simulink library "util_generic_model_lib"  (R2016b)
settings: Solver=ode45  StartTime=0.0  StopTime=10.0  RelTol=1e-3  EnableMultiTasking=on
undefined symbols (not defined in the file): abp_impeller_diameter, abp_impeller_speed2pwm, abp_nozzle_flap_count, abp_nozzle_flap_length, abp_nozzle_gear_ratio, abp_nozzle_intake_height, abp_nozzle_min_open_angle, abp_P_CG_B_B_error, abp_PM1_discharge_coeff, abp_pm1_impeller_orientation, abp_PM1_nozzle_orientations, abp_PM1_nozzle_widths, abp_PM1_P_nozzle_B_B, abp_pm1_zero_thrust_area, astrobee_time_step_size, bmp_PM1_impeller_orientation_error, bpm_imp_cmd_filt_den, bpm_imp_cmd_filt_num, bpm_imp_ctl_filt_n, bpm_imp_ctl_kd, bpm_imp_ctl_ki, bpm_imp_ctl_kp, bpm_imp_ctl_ts, bpm_imp_max_voltage, bpm_imp_motor_friction_coeff, bpm_imp_motor_r, bpm_imp_motor_speed_k, bpm_imp_motor_torque_k, bpm_imp_speed_filt_den, bpm_imp_speed_filt_num, bpm_impeller_inertia, bpm_impeller_inertia_error, bpm_impeller_init_speed, bpm_lookup_Cdp_data, bpm_lookup_totalarea_breakpoints, bpm_noise_on_flag, bpm_PM1_nozzle_discharge_coeff_error, bpm_PM1_nozzle_noise_feedback_gain, bpm_PM1_nozzle_thrust_noise_1s, bpm_PM1_P_nozzle_B_B_error, bpm_PM1_Q_nozzle2misaligned, bpm_PM1_randn_noise_seed, bpm_PM1_zero_thrust_area_error, bpm_sensor_delay, bpm_sensor_max, bpm_sensor_min, bpm_sensor_rand_seed, bpm_sensor_resolution, bpm_sensor_sf, bpm_sensor_sigma_u, bpm_sensor_sigma_v, bpm_servo_ctl_filt_n, bpm_servo_ctl_kd, bpm_servo_ctl_ki, bpm_servo_ctl_kp, bpm_servo_ctl_ts, bpm_servo_max_theta, bpm_servo_max_voltage, bpm_servo_min_theta, bpm_servo_motor_backlash_deadband ... (+45)
libraries: math_utils x8, simulink x4, vrlib x3, util_generic_model_lib x2
(part 2 of 2)

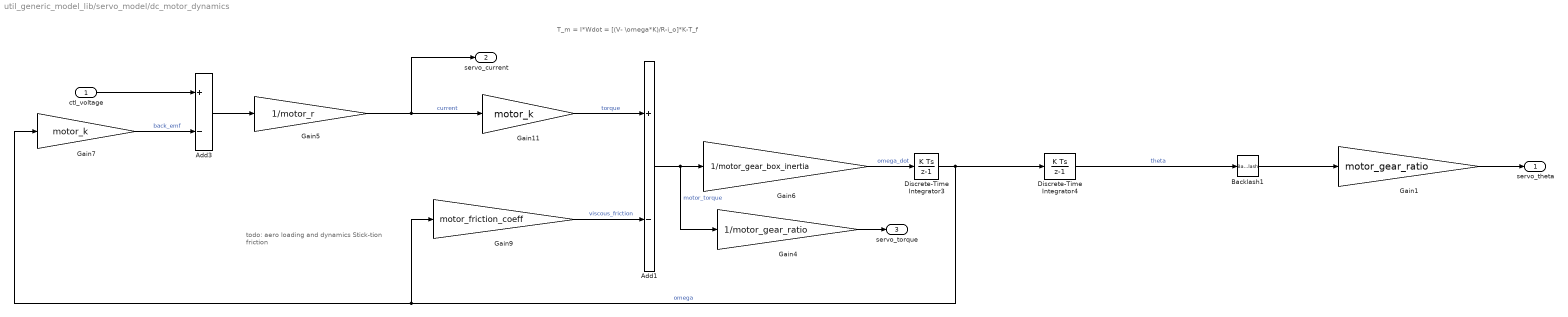
== system util_generic_model_lib/servo_model/dc_motor_dynamics ==
  note: todo:
      | aero loading and dynamics
      | Stick-tion friction
  note: T_m = I*Wdot = [(V- \omega*K)/R-i_o]*K-T_f
  ctl_voltage : Inport
  Add1 : Sum  Inputs=+-
  Add3 : Sum  Inputs=+-
  Backlash1 : Backlash  BacklashWidth=motor_backlash_deadband
      settings: AttributesFormatString=width: %<BacklashWidth>
  Discrete-Time Integrator3 : DiscreteIntegrator  InitialCondition=single(0)  SampleTime=-1  ICPrevOutput=DiscIntNeverNeededParam  ICPrevScaledInput=DiscIntNeverNeededParam
      settings: AttributesFormatString=IC: %<InitialCondition>
  Discrete-Time Integrator4 : DiscreteIntegrator  InitialCondition=servo_min_theta/motor_gear_ratio  SampleTime=-1  LimitOutput=on  UpperSaturationLimit=servo_max_theta/motor_gear_ratio  LowerSaturationLimit=servo_min_theta/motor_gear_ratio  ICPrevOutput=DiscIntNeverNeededParam  ICPrevScaledInput=DiscIntNeverNeededParam
      settings: AttributesFormatString=|
      | IC: %<InitialCondition>
      | max: %<UpperSaturationLimit>
      | min: %<LowerSaturationLimit>
  Gain1 : Gain  Gain=motor_gear_ratio
  Gain11 : Gain  Gain=motor_k
  Gain4 : Gain  Gain=1/motor_gear_ratio
  Gain5 : Gain  Gain=1/motor_r
  Gain6 : Gain  Gain=1/motor_gear_box_inertia
  Gain7 : Gain  Gain=motor_k
  Gain9 : Gain  Gain=motor_friction_coeff
  servo_theta : Outport
  servo_current : Outport  Port=2
  servo_torque : Outport  Port=3
  wires:
  Gain6/1 -> Discrete-Time Integrator3/1  "omega_dot"
  Gain7/1 -> Add3/2  "back_emf"
  Gain5/1 -> Gain11/1, servo_current/1  "current"
  Discrete-Time Integrator4/1 -> Backlash1/1  "theta"
  Discrete-Time Integrator3/1 -> Discrete-Time Integrator4/1, Gain7/1, Gain9/1  "omega"
  Backlash1/1 -> Gain1/1
  Gain1/1 -> servo_theta/1
  Add1/1 -> Gain4/1, Gain6/1  "motor_torque"
  Gain11/1 -> Add1/1  "torque"
  Gain9/1 -> Add1/2  "viscous_friction"
  Gain4/1 -> servo_torque/1
  ctl_voltage/1 -> Add3/1
  Add3/1 -> Gain5/1

== system util_generic_model_lib/servo_model/servo_controller ==
  command_PWM : Inport
  curr_servo_theta : Inport  Port=2
  Constant : Constant  Value=servo_pwm2angle_bias
  Discrete PID Controller : simulink/Continuous/PID Controller  Controller=PID  TimeDomain=Discrete-time  SampleTime=servo_ctl_ts  IntegratorMethod=Forward Euler  FilterMethod=Forward Euler  Form=Parallel  UseFilter=on  ControllerParametersSource=internal  P=servo_ctl_kp  I=servo_ctl_ki  D=servo_ctl_kd  N=servo_ctl_filt_n  InitialConditionSource=internal  InitialConditionForIntegrator=0  InitialConditionForFilter=0  ExternalReset=none  LimitOutput=on  UpperSaturationLimit=servo_max_voltage  LowerSaturationLimit=-servo_max_voltage  LinearizeAsGain=off  AntiWindupMode=clamping  Kb=1  TrackingMode=off  Kt=1  PParamMin=[]  PParamMax=[]  IParamMin=[]  IParamMax=[]  DParamMin=[]  DParamMax=[]  NParamMin=[]  NParamMax=[]  KbParamMin=[]  KbParamMax=[]  KtParamMin=[]  KtParamMax=[]  POutMin=[]  POutMax=[]  IOutMin=[]  IOutMax=[]  DOutMin=[]  DOutMax=[]  NOutMin=[]  NOutMax=[]  KbOutMin=[]  KbOutMax=[]  KtOutMin=[]  KtOutMax=[]  IntegratorOutMin=[]  IntegratorOutMax=[]  FilterOutMin=[]  FilterOutMax=[]  SumOutMin=[]  SumOutMax=[]  SumI1OutMin=[]  SumI1OutMax=[]  SumI2OutMin=[]  SumI2OutMax=[]  SumI3OutMin=[]  SumI3OutMax=[]  SumDOutMin=[]  SumDOutMax=[]  SaturationOutMin=[]  SaturationOutMax=[]  IntegratorContinuousStateAttributes=''  IntegratorStateMustResolveToSignalObject=off  IntegratorRTWStateStorageClass=Auto  FilterContinuousStateAttributes=''  FilterStateMustResolveToSignalObject=off  FilterRTWStateStorageClass=Auto  DifferentiatorICPrevScaledInput=0  DifferentiatorOutMin=[]  DifferentiatorOutMax=[]
      settings: AttributesFormatString=|
      | Kp: %<P>
      | Ki: %<I>
      | Kd: %<D>
      | NFilt: %<N>
      | Ts: %<SampleTime>
      | 
      | Min: %<LowerSaturationLimit>
      | Max: %<UpperSaturationLimit>
  Gain : Gain  Gain=servo_pwm2angle
  Sum : Sum
  Sum1 : Sum  Inputs=+-
  motor_ctl_voltage : Outport
  wires:
  Gain/1 -> Sum1/1  "cmd_servo_theta"
  curr_servo_theta/1 -> Sum1/2
  Discrete PID Controller/1 -> motor_ctl_voltage/1
  Constant/1 -> Sum/2
  command_PWM/1 -> Sum/1
  Sum1/1 -> Discrete PID Controller/1
  Sum/1 -> Gain/1

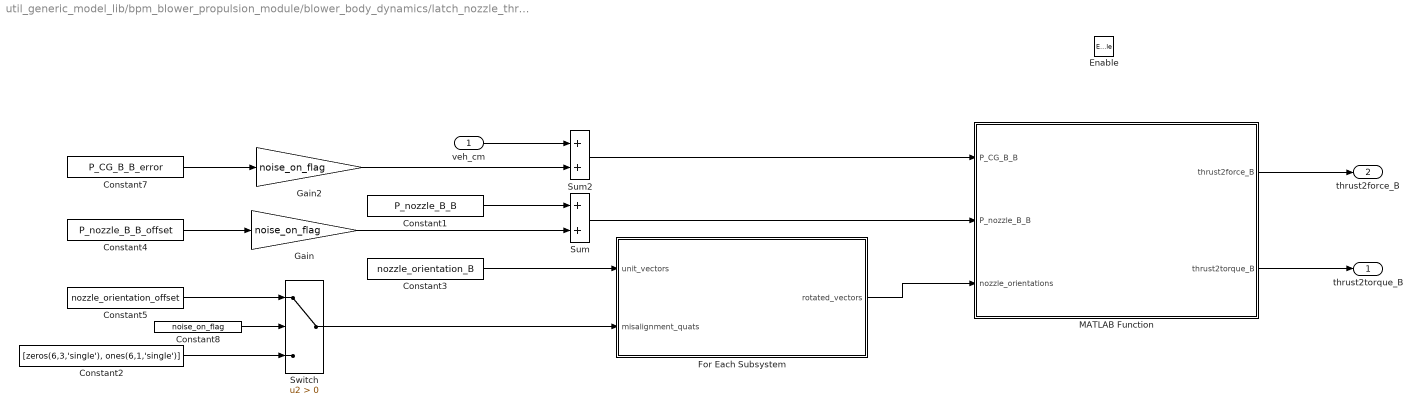
== system util_generic_model_lib/bpm_blower_propulsion_module/blower_body_dynamics/latch_nozzle_thrust_matricies ==
  veh_cm : Inport
  Enable : EnablePort  ZeroCross=off
  Constant1 : Constant  Value=P_nozzle_B_B
  Constant2 : Constant  Value=[zeros(6,3,'single'), ones(6,1,'single')]
  Constant3 : Constant  Value=nozzle_orientation_B
  Constant4 : Constant  Value=P_nozzle_B_B_offset
  Constant5 : Constant  Value=nozzle_orientation_offset
  Constant7 : Constant  Value=P_CG_B_B_error  VectorParams1D=off
  Constant8 : Constant  Value=noise_on_flag
  For Each Subsystem : Subsystem  TreatAsAtomicUnit=on
  Gain : Gain  Gain=noise_on_flag
  Gain2 : Gain  Gain=noise_on_flag
  MATLAB Function : MATLAB Function  TreatAsAtomicUnit=on
  Sum : Sum
  Sum2 : Sum
  Switch : Switch  Criteria=u2 > Threshold
  thrust2torque_B : Outport
  thrust2force_B : Outport  Port=2
  wires:
  Constant8/1 -> Switch/2
  Constant2/1 -> Switch/3
  Switch/1 -> For Each Subsystem/2(misalignment_quats)
  Gain/1 -> Sum/2
  Constant5/1 -> Switch/1
  Constant4/1 -> Gain/1
  Sum/1 -> MATLAB Function/2(P_nozzle_B_B)
  MATLAB Function/2(thrust2torque_B) -> thrust2torque_B/1
  MATLAB Function/1(thrust2force_B) -> thrust2force_B/1
  Constant3/1 -> For Each Subsystem/1(unit_vectors)
  Constant1/1 -> Sum/1
  For Each Subsystem/1(rotated_vectors) -> MATLAB Function/3(nozzle_orientations)
  Gain2/1 -> Sum2/2
  Constant7/1 -> Gain2/1
  Sum2/1 -> MATLAB Function/1(P_CG_B_B)
  veh_cm/1 -> Sum2/1

== system util_generic_model_lib/bpm_blower_propulsion_module/blower_body_dynamics/latch_nozzle_thrust_matricies/For Each Subsystem ==
  unit_vectors : Inport  Partition=on  PartitionDimension=1  PartitionWidth=1
  misalignment_quats : Inport  Port=2  Partition=on  PartitionDimension=1  PartitionWidth=1
  For Each : ForEach  DisableCoverage=on  IndexMode=One-based
  Reshape : Reshape  OutputDimensionality=Row vector (2-D)
  Reshape1 : Reshape
  rotate_vec_A2B : math_utils/rotate_vec_A2B  SystemSampleTime=-1
  rotated_vectors : Outport  ConcatenationDimension=1
  wires:
  Reshape/1 -> rotated_vectors/1
  unit_vectors/1 -> Reshape1/1
  misalignment_quats/1 -> rotate_vec_A2B/2
  rotate_vec_A2B/1 -> Reshape/1
  Reshape1/1 -> rotate_vec_A2B/1

== matlab function util_generic_model_lib/bpm_blower_propulsion_module/blower_body_dynamics/latch_nozzle_thrust_matricies/MATLAB Function ==
  data: P_CG_B_B input; P_nozzle_B_B input; nozzle_orientations input; thrust2force_B output; thrust2torque_B output
function [thrust2force_B, thrust2torque_B] = calc_thrust_matricies(P_CG_B_B, P_nozzle_B_B, nozzle_orientations)
%#codegen

%NOTE: if number of nozzles change, must change this hard coded '6' below
nozzle_moment_arm       = P_nozzle_B_B - repmat(P_CG_B_B,6,1);                 %[m] Distance from nozzles to CG

thrust2torque_B         = -cross(nozzle_moment_arm, nozzle_orientations,2)';   %[-] Converts a nozzle thrust into resulting body torques
thrust2force_B          = -nozzle_orientations';                               %[-] Converts a nozzle thrust into resulting body forces
end
